simulink model "Model"  (R2023b)
settings: Solver=VariableStepAuto  StartTime=0.0  StopTime=10  RelTol=1e-3
values from neighbouring files (symbols this model uses):
  f0 = 50e6    (= 50000000)    [Noise_sim_script.m]    (also in fit_ecs_phase_noise.m; oscilator.m = 10000000)
  pn_filter_b = 1    [Noise_sim_script.m]
  T_bp = [-40 -30 -20 -10 0 10 20 30           40 50 60 70 80 90 100 105]    [initial_oscillator_temp_model.m]
  Ts_noise = 1/fs_noise    (= 2e-06)    [Noise_sim_script.m]
  yT_typ_ppb = [-25 -20 -14 -9 -5 -2 2 7                 12 15 15 13 10 7 3 0]    [initial_oscillator_temp_model.m]
libraries: simulink x4
settings Model: Creator=Admin  LastModifiedBy=Admin

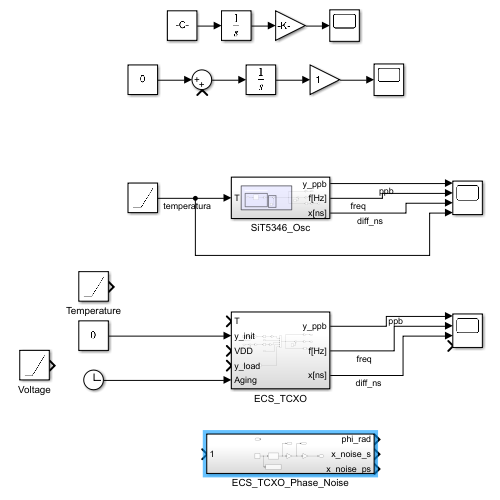
[thumbnail: Simulink's stored preview of the top-level diagram]
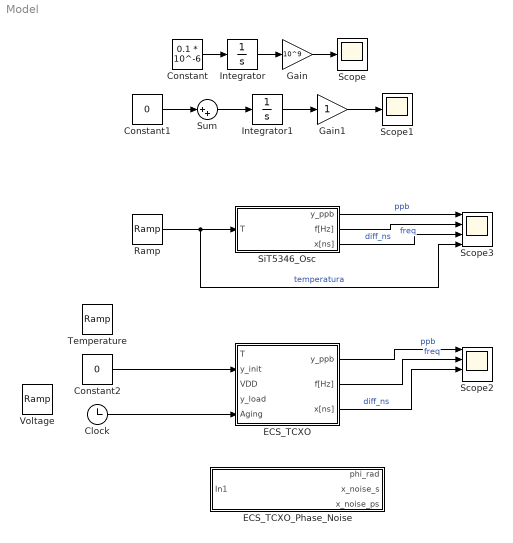
== system Model ==
  Clock : Clock
  Constant : Constant  Value=0.1 * 10^-6
  Constant1 : Constant  Value=0
  Constant2 : Constant  Value=0
  ECS_TCXO : Subsystem
  ECS_TCXO_Phase_Noise : Subsystem
  Gain : Gain  Gain=10^9
  Gain1 : Gain
  Integrator : Integrator
  Integrator1 : Integrator
  Ramp : simulink/Sources/Ramp  slope=0.5/60  start=0  InitialOutput=25
  Scope : Scope
  Scope1 : Scope
  Scope2 : Scope  NumInputPorts=4
  Scope3 : Scope  NumInputPorts=4
  SiT5346_Osc : Subsystem
  Sum : Sum  Inputs=|++
  Temperature : simulink/Sources/Ramp  slope=0.5/60  start=0  InitialOutput=25
  Voltage : simulink/Sources/Ramp  slope=0.165/100  start=0  InitialOutput=3.3
  wires:
  Constant/1 -> Integrator/1
  Integrator/1 -> Gain/1
  Gain/1 -> Scope/1
  Integrator1/1 -> Gain1/1
  Sum/1 -> Integrator1/1
  Constant1/1 -> Sum/1
  Gain1/1 -> Scope1/1
  SiT5346_Osc/2(f[Hz]) -> Scope3/2  "freq"
  SiT5346_Osc/1(y_ppb) -> Scope3/1  "ppb"
  SiT5346_Osc/3(x[ns]) -> Scope3/3  "diff_ns"
  Ramp/1 -> Scope3/4, SiT5346_Osc/1(T)  "temperatura"
  ECS_TCXO/2(f[Hz]) -> Scope2/2  "freq"
  ECS_TCXO/3(x[ns]) -> Scope2/3  "diff_ns"
  ECS_TCXO/1(y_ppb) -> Scope2/1  "ppb"
  Constant2/1 -> ECS_TCXO/2(y_init)
  Clock/1 -> ECS_TCXO/5(Aging)

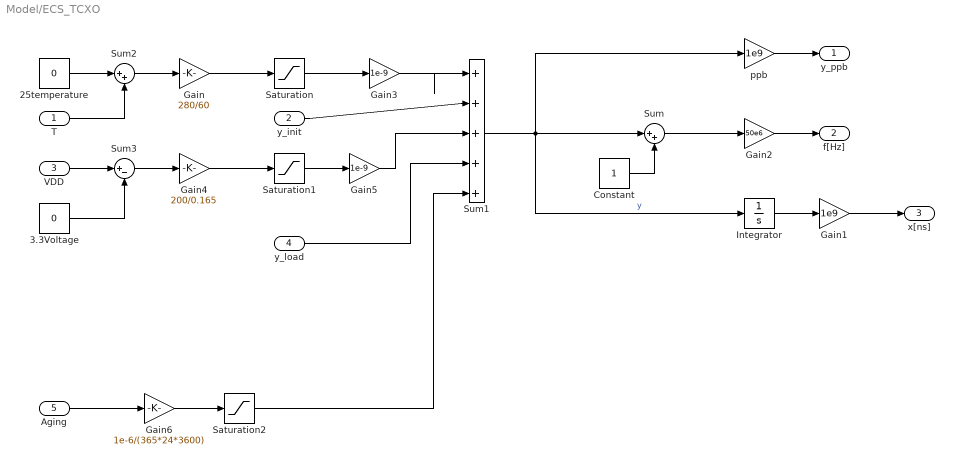
== system Model/ECS_TCXO ==
  T : Inport
  y_init : Inport  Port=2
  VDD : Inport  Port=3
  y_load : Inport  Port=4
  Aging : Inport  Port=5
  25temperature : Constant  Value=0
  3.3Voltage : Constant  Value=0
  Constant : Constant
  Gain : Gain  Gain=280/60
  Gain1 : Gain  Gain=1e9
  Gain2 : Gain  Gain=50e6
  Gain3 : Gain  Gain=1e-9
  Gain4 : Gain  Gain=200/0.165
  Gain5 : Gain  Gain=1e-9
  Gain6 : Gain  Gain=1e-6/(365*24*3600)
  Integrator : Integrator
  Saturation : Saturate  UpperLimit=280  LowerLimit=-280
  Saturation1 : Saturate  UpperLimit=200  LowerLimit=-200
  Saturation2 : Saturate  UpperLimit=1e-6  LowerLimit=-1e-6
  Sum : Sum  Inputs=|++
  Sum1 : Sum  Inputs=|+++++
  Sum2 : Sum  Inputs=|++
  Sum3 : Sum  Inputs=|+-
  ppb : Gain  Gain=1e9
  y_ppb : Outport
  f[Hz] : Outport  Port=2
  x[ns] : Outport  Port=3
  wires:
  ppb/1 -> y_ppb/1
  Integrator/1 -> Gain1/1
  Gain1/1 -> x[ns]/1
  Sum1/1 -> ppb/1, Integrator/1, Sum/1  "y"
  Gain2/1 -> f[Hz]/1
  Sum/1 -> Gain2/1
  Constant/1 -> Sum/2
  y_init/1 -> Sum1/2
  y_load/1 -> Sum1/4
  T/1 -> Sum2/2
  25temperature/1 -> Sum2/1
  Sum2/1 -> Gain/1
  Gain/1 -> Saturation/1
  Saturation/1 -> Gain3/1
  Gain3/1 -> Sum1/1
  VDD/1 -> Sum3/1
  3.3Voltage/1 -> Sum3/2
  Sum3/1 -> Gain4/1
  Gain4/1 -> Saturation1/1
  Saturation1/1 -> Gain5/1
  Gain5/1 -> Sum1/3
  Aging/1 -> Gain6/1
  Gain6/1 -> Saturation2/1
  Saturation2/1 -> Sum1/5

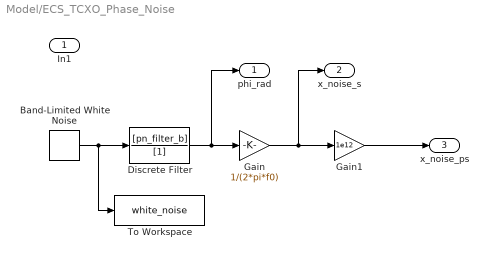
== system Model/ECS_TCXO_Phase_Noise ==
  In1 : Inport
  Band-Limited White Noise : simulink/Sources/Band-Limited White Noise  Cov=[1]  Ts=Ts_noise  seed=[12345]
  Discrete Filter : DiscreteFilter  Numerator=[pn_filter_b]  Denominator=[1]
  Gain : Gain  Gain=1/(2*pi*f0)
  Gain1 : Gain  Gain=1e12
  To Workspace : ToWorkspace  VariableName=white_noise  SampleTime=-1
  phi_rad : Outport
  x_noise_s : Outport  Port=2
  x_noise_ps : Outport  Port=3
  wires:
  Band-Limited White Noise/1 -> To Workspace/1, Discrete Filter/1
  Discrete Filter/1 -> phi_rad/1, Gain/1
  Gain/1 -> x_noise_s/1, Gain1/1
  Gain1/1 -> x_noise_ps/1

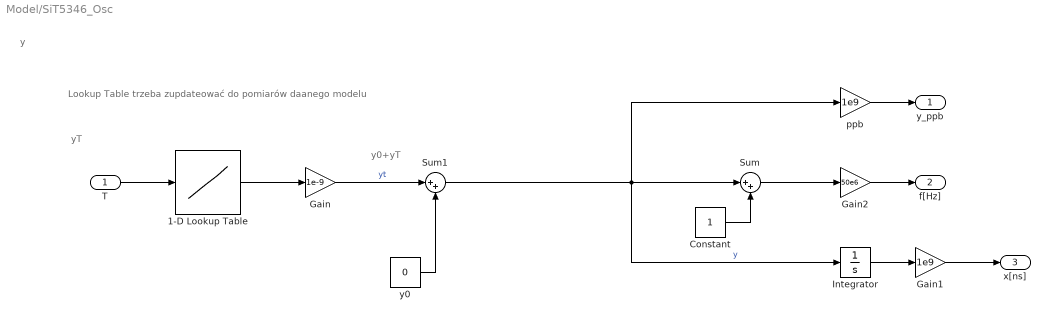
== system Model/SiT5346_Osc ==
  note: Lookup Table trzeba zupdateować do pomiarów daanego modelu
  note: y0+yT
  note: y
  note: yT
  T : Inport
  1-D Lookup Table : Lookup_n-D  NumberOfTableDimensions=1  BreakpointsForDimension1=T_bp  Table=yT_typ_ppb  InternalRulePriority=Speed  RndMeth=Simplest
  Constant : Constant
  Gain : Gain  Gain=1e-9
  Gain1 : Gain  Gain=1e9
  Gain2 : Gain  Gain=50e6
  Integrator : Integrator
  Sum : Sum  Inputs=|++
  Sum1 : Sum  Inputs=|++
  ppb : Gain  Gain=1e9
  y0 : Constant  Value=0
  y_ppb : Outport
  f[Hz] : Outport  Port=2
  x[ns] : Outport  Port=3
  wires:
  T/1 -> 1-D Lookup Table/1
  y0/1 -> Sum1/2
  ppb/1 -> y_ppb/1
  Integrator/1 -> Gain1/1
  Gain1/1 -> x[ns]/1
  Sum1/1 -> Sum/1, Integrator/1, ppb/1  "y"
  1-D Lookup Table/1 -> Gain/1
  Gain/1 -> Sum1/1  "yt"
  Gain2/1 -> f[Hz]/1
  Sum/1 -> Gain2/1
  Constant/1 -> Sum/2
